simulink model "output7"  (R2018a)
settings: Solver=FixedStepAuto  StartTime=0.0  StopTime=10.0  FixedStep=1  RelTol=1e-3
undefined symbols (not defined in the file or in its folder): Ad_blue_level, Ad_blue_temp
settings Model: DataDictionary=output7_data.sldd  Creator=Home  LastModifiedBy=Home

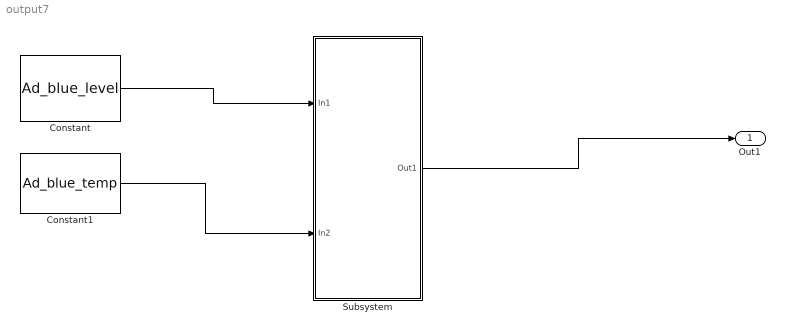
== system output7 ==
  Constant : Constant  Value=Ad_blue_level
  Constant1 : Constant  Value=Ad_blue_temp
  Subsystem : Subsystem
  Out1 : Outport
  wires:
  Constant/1 -> Subsystem/1(In1)
  Constant1/1 -> Subsystem/2(In2)
  Subsystem/1(Out1) -> Out1/1

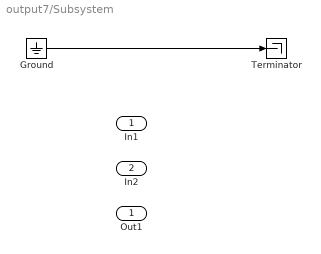
== system output7/Subsystem ==
  In1 : Inport
  In2 : Inport  Port=2
  Ground : Ground
  Terminator : Terminator
  Out1 : Outport
  wires:
  Ground/1 -> Terminator/1
